simulink model "crankshaft_models"  (R2022b)
settings: Solver=FixedStepAuto  StartTime=0.0  StopTime=10.0  FixedStep=0.0001  RelTol=1e-3
settings Model: Creator=saidb  LastModifiedBy=saidb

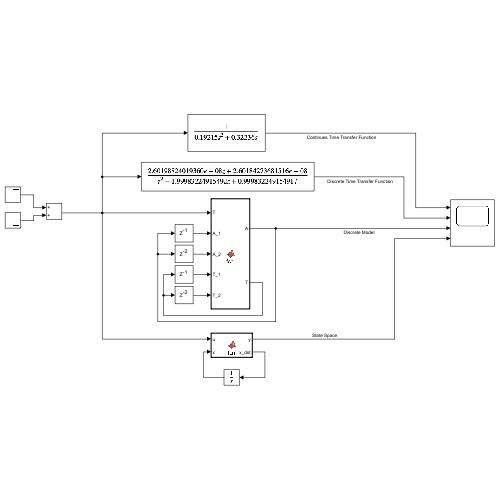
[thumbnail: Simulink's stored preview of the top-level diagram]
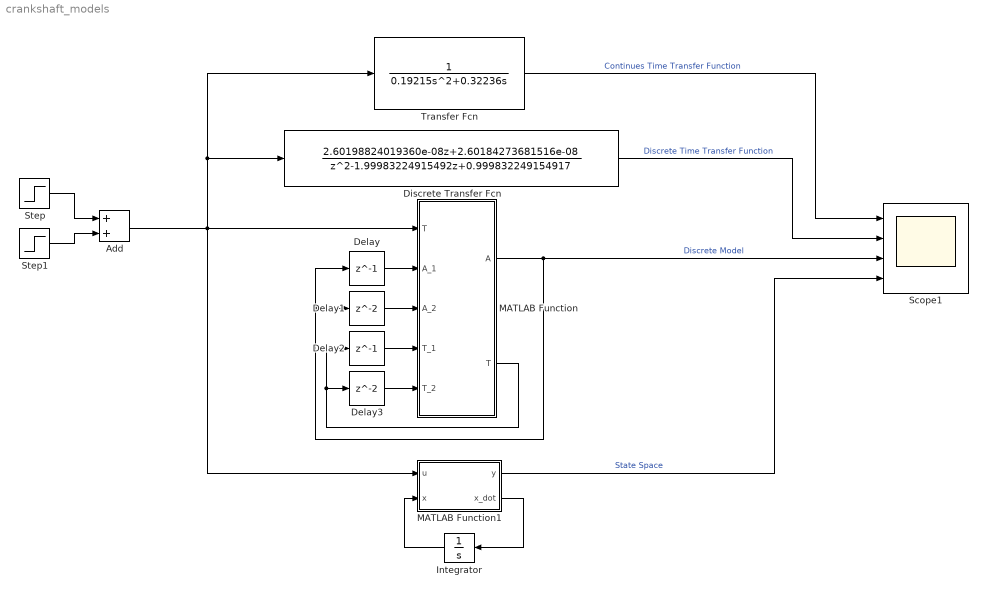
== system crankshaft_models ==
  Add : Sum
  Delay : Delay  DelayLength=1
  Delay1 : Delay
  Delay2 : Delay  DelayLength=1
  Delay3 : Delay
  Discrete Transfer Fcn : DiscreteTransferFcn  Numerator=[0,2.60198824019360e-08,2.60184273681516e-08]  Denominator=[1,-1.99983224915492,0.999832249154917]
  Integrator : Integrator  InitialCondition=[0;0]
  MATLAB Function : MATLAB Function  TreatAsAtomicUnit=on
  MATLAB Function1 : MATLAB Function  TreatAsAtomicUnit=on
  Scope1 : Scope  NumInputPorts=4
  Step : Step  Time=0  After=10  SampleTime=0
  Step1 : Step  Time=2  After=-10  SampleTime=0
  Transfer Fcn : TransferFcn  Denominator=[0.19215 0.32236 0]
  wires:
  Add/1 -> MATLAB Function1/1(u), Discrete Transfer Fcn/1, Transfer Fcn/1, MATLAB Function/1("T ")
  Step/1 -> Add/1
  Integrator/1 -> MATLAB Function1/2(x)
  MATLAB Function1/1(y) -> Scope1/4  "State Space"
  Delay2/1 -> MATLAB Function/4(T_1)
  MATLAB Function/2(T) -> Delay3/1, Delay2/1
  Transfer Fcn/1 -> Scope1/1  "Continues Time Transfer Function"
  MATLAB Function1/2(x_dot) -> Integrator/1
  Step1/1 -> Add/2
  Discrete Transfer Fcn/1 -> Scope1/2  "Discrete Time Transfer Function"
  MATLAB Function/1(A) -> Delay1/1, Delay/1, Scope1/3  "Discrete Model"
  Delay3/1 -> MATLAB Function/5(T_2)
  Delay1/1 -> MATLAB Function/3(A_2)
  Delay/1 -> MATLAB Function/2(A_1)

== matlab function crankshaft_models/MATLAB Function1 ==
  data: y output; u input; x input; x_dot output
function [y, x_dot] = fcn(u, x)

I = 0.19215;
c = 0.32236;
k = 0;

A = [0 1;
    -k/I -c/I];
B = [0;
    1/I];
C = [1 0];
D = 0;

x_dot = A * x + B * u;
y = C * x + D * u;

== matlab function crankshaft_models/MATLAB Function ==
  data: T input; A_1 input; A_2 input; T_1 input; T_2 input; A output; T output
function [A, T] = fcn(T, A_1, A_2, T_1, T_2)

A = (2.601988240193600e-08) * T_1 + (2.601842736815161e-08) * ...
    T_2 + (1.999832249154917) * A_1 - (0.999832249154917) * A_2;
